simulink model "PSO_thuc_nghiem"  (R2021a)
settings: Solver=VariableStepAuto  StartTime=0.0  StopTime=10  RelTol=1e-3
InitFcn:
  | mc=0.5;
  | g=9.81;
  | n1=5;n2=1;
  | 
  | L2=0.5;
  | m1=2;
  | m2=mc;
  | m=5;
  | %Bo input shaping
  | alpha = (1/L1 + 1/L2)*(m1+m2)/m1;
  | beta = (((m1+m2)/m1)^2)*((1/L1 + 1/L2)^2) - 4*(m1+m2)/(m1*L1*L2);
  | w1 = sqrt(g*(alpha - sqrt(beta))/2);
  | w2 = sqrt(g*(alpha + sqrt(beta))/2);
  | damping_ratio = 0;
  | wd1 = w1*sqrt(1-damping_ratio^2);
  | wd2 = w2*sqrt(1-damping_ratio^2);
  | k = exp(damping_ratio*pi/sqrt(1-damping_ratio^2));
  | 
  | %ETM4_1
  | m_etm4_1 = 0.1;
  | I_etm4_1 = (1+m_etm4_1)*k*k/(k^2 + (1+m_etm4_1)*(k^(4/3)+k^(2/3)) + m_etm4_1);
  | A1_etm4_1 = I_etm4_1/(1+m_etm4_1);
  | A2_etm4_1 = I_etm4_1/(k^(2/3));
  | A3_etm4_1 = I_etm4_1/(k^(4/3));
  | A4_etm4_1 = m_etm4_1*I_etm4_1/((1+m_etm4_1)*(k^2));
  | t1_etm4_1 = (2*pi/3)/wd1;
  | t2_etm4_1 = (4*pi/3)/wd1;
  | t3_etm4_1 = 2*pi/wd1;
  | %ETM4_2
  | m_etm4_2 = 0.1;
  | I_etm4_2 = (1+m_etm4_2)*k*k/(k^2 + (1+m_etm4_2)*(k^(4/3)+k^(2/3)) + m_etm4_2);
  | A1_etm4_2 = I_etm4_2/(1+m_etm4_2);
  | A2_etm4_2 = I_etm4_2/(k^(2/3));
  | A3_etm4_2 = I_etm4_2/(k^(4/3));
  | A4_etm4_2 = m_etm4_2*I_etm4_2/((1+m_etm4_2)*(k^2));
  | t1_etm4_2 = (2*pi/3)/wd2;
  | t2_etm4_2 = (4*pi/3)/wd2;
  | t3_etm4_2 = 2*pi/wd2;
values from neighbouring files (symbols this model uses):
  l_ini = L    [PSO_ZVD.m]
  particle = repmat(empty_particle, nPop, 1)    [PSO16_12.m]    (also in PSO_ZVD.m)
undefined symbols (not defined in the file or in its folder): b0, b1, i, Kd, Kd1, Kp, Kp1, l, l1, l11, l2, l21, l3, l31, l_ref, li, M2, x_ref, xi
libraries: neural x70, simulink_extras x11, simulink x5
(part 15 of 25)

== matlab function PSO_thuc_nghiem/Hieu/Model_Baocao/Crane ==
  data: d1x input; l input; d1l input; the input; dx1 output; d1the input; Fx input; Fl input; dx2 output; dx3 output; dx4 output; dx5 output; dx6 output; bc input; mp input
function [dx1,dx2,dx3,dx4,dx5,dx6] = fcn(d1x,l,d1l,the,d1the,Fx,Fl,bc,mp)
 mt =5; mh =2; bt =20; br =50;  g =9.81;

dx1 = d1x;
dx2 = (Fx*l*mh + Fx*l*mp - Fl*l*mp*sin(the) + bc*d1the*mh*cos(the) + bc*d1the*mp*cos(the) - d1the^2*l^2*mp^2*sin(the) + d1x^2*l^2*mp^2*sin(the) - bt*d1x*l*mh - bt*d1x*l*mp + d1x^2*l^2*mh*mp*sin(the) + br*d1l*l*mp*sin(the) + g*l*mh*mp*cos(the)*sin(the))/(l*(mh*mp + mh*mt + mp*mt - mp^2*cos(the)^2 - mp^2*sin(the)^2 + mp^2 - mh*mp*cos(the)^2));
%dx2= -(bt*x2*mc - ml*ut - mc*ul*sin(x5) - mc*ut + bt*x2*ml - x6^2*x3*mc^2*sin(x5) + br*x4*mc*sin(x5) + Dt*x6*mc^2*cos(x5) + x6^2*x3*mc*ml*sin(x5) + g*mc*ml*cos(x5)*sin(x5) + Dt*x6*mc*ml*cos(x5))/(mc*ml + mc*mt + ml*mt - mc^2*cos(x5)^2 - mc^2*sin(x5)^2 + mc^2 - mc*ml*cos(x5)^2);
 
dx3 = d1l;
dx4 = -(d1x^2*l^2*mp^2*sin(the)^2 - Fl*l*mt - d1the^2*l^2*mp^2 - Fl*l*mp + g*l*mp^2*cos(the)^3 + Fx*l*mp*sin(the) + Fl*l*mp*cos(the)^2 - d1the^2*l^2*mp*mt - g*l*mp^2*cos(the) + d1the^2*l^2*mp^2*cos(the)^2 + br*d1l*l*mp + br*d1l*l*mt + g*l*mp^2*cos(the)*sin(the)^2 - br*d1l*l*mp*cos(the)^2 + bc*d1the*mp*cos(the)*sin(the) - g*l*mp*mt*cos(the) - bt*d1x*l*mp*sin(the))/(l*(mh*mp + mh*mt + mp*mt - mp^2*cos(the)^2 - mp^2*sin(the)^2 + mp^2 - mh*mp*cos(the)^2));
%dx4 = -(mc*ul*cos(x5)^2 - mt*ul - mc*ut*sin(x5) - 2*x6^2*x3*mc^2 - g*mc^2*cos(x5) - mc*ul + br*x4*mc + br*x4*mt + g*mc^2*cos(x5)^3 - 2*x6^2*x3*mc*mt - g*mc*mt*cos(x5) + bt*x2*mc*sin(x5) + 2*x6^2*x3*mc^2*cos(x5)^2 + x6^2*x3*mc^2*sin(x5)^2 + g*mc^2*cos(x5)*sin(x5)^2 - br*x4*mc*cos(x5)^2 + Dt*x6*mc^2*cos(x5)*sin(x5))/(mc*ml + mc*mt + ml*mt - mc^2*cos(x5)^2 - mc^2*sin(x5)^2 + mc^2 - mc*ml*cos(x5)^2);
dx5 = d1the;
dx6 = -(bc*d1the*mp^2 + bc*d1the*mh*mp + bc*d1the*mh*mt + bc*d1the*mp*mt - bc*d1the*mp^2*sin(the)^2 - g*l*mp^3*sin(the)^3 + 2*d1l*d1the*l*mp^3 + Fx*l*mp^2*cos(the) + g*l*mp^3*sin(the) - g*l*mp^3*cos(the)^2*sin(the) - bt*d1x*l*mp^2*cos(the) + g*l*mh*mp^2*sin(the) + g*l*mp^2*mt*sin(the) - d1the^2*l^2*mp^3*cos(the)*sin(the) + d1x^2*l^2*mp^3*cos(the)*sin(the) - 2*d1l*d1the*l*mp^3*cos(the)^2 - Fl*l*mp^2*cos(the)*sin(the) - 2*d1l*d1the*l*mp^3*sin(the)^2 + Fx*l*mh*mp*cos(the) + 2*d1l*d1the*l*mh*mp^2 + 2*d1l*d1the*l*mp^2*mt - 2*d1l*d1the*l*mh*mp^2*cos(the)^2 + br*d1l*l*mp^2*cos(the)*sin(the) - bt*d1x*l*mh*mp*cos(the) + g*l*mh*mp*mt*sin(the) + 2*d1l*d1the*l*mh*mp*mt + d1x^2*l^2*mh*mp^2*cos(the)*sin(the))/(l^2*mp*(mh*mp + mh*mt + mp*mt - mp^2*cos(the)^2 - mp^2*sin(the)^2 + mp^2 - mh*mp*cos(the)^2));
%dx6 = -(g*mc^2*sin(x5) - ml*ut*cos(x5) - mc*ut*cos(x5) + Dt*x6*mc^2 - g*mc^2*sin(x5)^3 + 2*x4*x6*mc^2 - mc*ul*cos(x5)*sin(x5) + 2*x4*x6*mc*ml + 2*x4*x6*mc*mt + 2*x4*x6*ml*mt - Dt*x6*mc^2*sin(x5)^2 - 2*x4*x6*mc^2*cos(x5)^2 - 2*x4*x6*mc^2*sin(x5)^2 + bt*x2*mc*cos(x5) + bt*x2*ml*cos(x5) + g*mc*ml*sin(x5) + g*mc*mt*sin(x5) + g*ml*mt*sin(x5) - g*mc^2*cos(x5)^2*sin(x5) + Dt*x6*mc*ml + Dt*x6*mc*mt + Dt*x6*ml*mt - x6^2*x3*mc^2*cos(x5)*sin(x5) - 2*x4*x6*mc*ml*cos(x5)^2 + br*x4*mc*cos(x5)*sin(x5) + x6^2*x3*mc*ml*cos(x5)*sin(x5))/(x3*(mc*ml + mc*mt + ml*mt - mc^2*cos(x5)^2 - mc^2*sin(x5)^2 + mc^2 - mc*ml*cos(x5)^2));
